simulink model "APFC_finalmodel"  (R2024b)
settings: Solver=VariableStepAuto  StartTime=0.0  StopTime=50  RelTol=1e-3
libraries: spsBreakerLib x7, spsSeriesRLCLoadLib x7, spsRMSLib x2, spsACVoltageSourceLib x1, spsCurrentMeasurementLib x1, spsVoltageMeasurementLib x1, spsMeanLib x1, spsPowerLib x1, sps_lib x1
settings Model: Creator=VICTUS  LastModifiedBy=niranjan

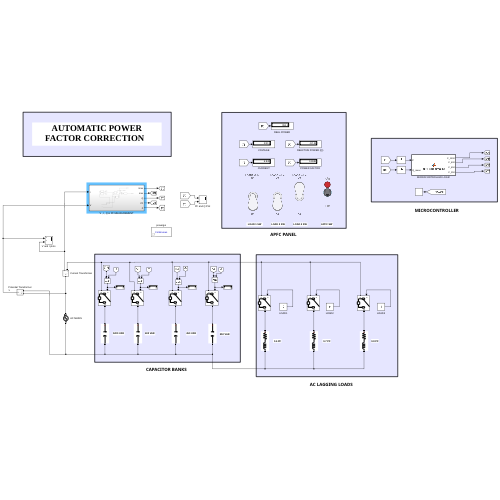
[thumbnail: Simulink's stored preview of the top-level diagram]
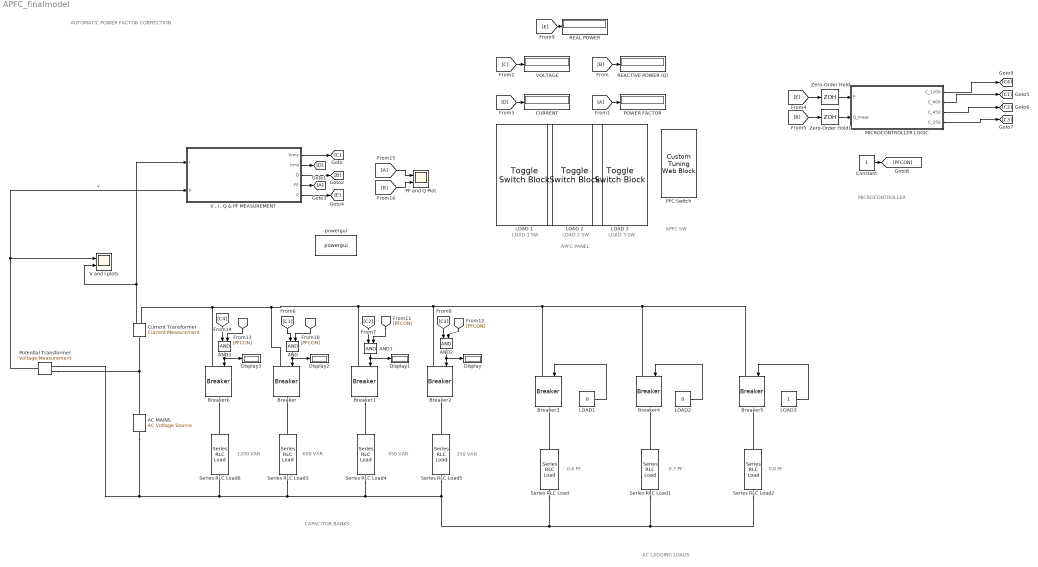
== system APFC_finalmodel ==
  note: AUTOMATIC POWER FACTOR CORRECTION
  note: CAPACITOR BANKS
  note: AC LAGGING LOADS
  note: 1200 VAR
  note: 600 VAR
  note: 450 VAR
  note: 350 VAR
  note: 0.6 PF
  note: 0.7 PF
  note: 0.8 PF
  note: MICROCONTROLLER
  note: APFC SW
  note: LOAD 3 SW
  note: LOAD 2 SW
  note: LOAD 1 SW
  note: APFC PANEL
  AC MAINS : spsACVoltageSourceLib/AC Voltage Source  Amplitude=325.27  Phase=0  Frequency=50  SampleTime=0  Measurements=None  BusType=swing  Pref=10e3  Qref=0  Qmin=-inf  Qmax=+inf
  AND{,1..3} (4 alike) : Logic  AllPortsSameDT=off  OutDataTypeStr=boolean
  Breaker{,1..6} (7 alike) : spsBreakerLib/Breaker  InitialState=0  SwitchingTimes="[1/60  5/60]"  External=on  BreakerResistance=0.01  SnubberResistance=1e6  SnubberCapacitance=inf  Measurements=None  MoreParameters=on  NoBreakLoop=off
  CURRENT : Display
  Constant : Constant
  Current Transformer : spsCurrentMeasurementLib/Current Measurement  PhasorSimulation=off  OutputType=Complex  PSBequivalent=0
  Display{,1..3} (4 alike) : Display
  From1 : From
  From15 : From
  Goto3 : Goto
  LOAD 1 : ToggleSwitchBlock
      settings: Values={{'Off', 'On'}, [0 1]}
  LOAD 2 : ToggleSwitchBlock
      settings: Values={{'Off', 'On'}, [0 1]}
  LOAD 3 : ToggleSwitchBlock
      settings: Values={{'Off', 'On'}, [0 1]}
  LOAD1 : Constant  Value=0
  LOAD2 : Constant  Value=0
  LOAD3 : Constant
  MICROCONTROLLER LOGIC : MATLAB Function  TreatAsAtomicUnit=on
  PF and Q Plot : Scope  NumInputPorts=2
  PFC Switch : CustomTuningWebBlock  LabelPosition=Hide  ShowInitialText=on  Configuration="{\"components\":[{\"name\":\"CustomSwitchStateComponent\",\"settings\":{\"position\":[0,0,1,1],\"showAllLabels\":1,\"states\":[{\"HitRegion\":{\"position\":[0.5,0,1,0.5]},\"Image\":{\"position\":[0,0.24928571428571428,0.5014285714285714,1],\"size\":[0.5014285714285714,1],\"src\":\"data:image\\/svg+xml;base64,PHN2ZyB4bWxucz0iaHR0cDovL3d3dy53My5vcmcvMjAwMC9zdmciIHhtbG5zOnhsaW5rPSJodHRwOi8vd3d3LnczLm9yZy8xOTk5L3hsaW5rIiB2aWV3Qm94PSIwIDAgMzguMDQgMTUwIj48ZGVmcz48c3R5bGU+LmNscy0xe2ZpbGw6dXJsKCNyYWRpYWwtZ3JhZGllbnQpO30uY2xzLTJ7ZmlsbDp1cmwoI3JhZGlhbC1ncmFkaWVudC0yKTt9LmNscy0ze2ZpbGw6dXJsKCNXaGl0ZV9CbGFjayk7fS5jbHMtNHtmaWxsOnVybCgjcmFkaWFsLWdyYWRpZW50LTMpO30uY2xzLTV7ZmlsbDojNWI1YjViO30uY2xzLTZ7ZmlsbDp1cmwoI3Jh ...(+3556 chars)\",\"srcOrientation\":\"Right\"},\"Label\":{\"color\":[0.5019607843137255,0.5019607843137255,0.5019607843137255],\"icon\":{\"size\":[0,0],\"src\":[],\"srcOrientation\":\"Right\"},\"iconOffset\":0,\"iconPlacement\":\"left\",\"opacity\":1,\"position\":[0.92,0.5],\"show\":true,\"text\":{\"content\":\"Off\",\"font\":\"Helvetica\"}},\"Value\":0},{\"HitRegion\":{\"position\":[0,0,1,0.5]},\"Image\":{\"position\":[0,0.24928571428571428,0.5014285714285714,1],\"size\":[0.5014285714285714,1],\"src\":\"data:image\\/svg+xml;base64,PHN2ZyB4bWxucz0iaHR0cDovL3d3dy53My5vcmcvMjAwMC9zdmciIHhtbG5zOnhsaW5rPSJodHRwOi8vd3d3LnczLm9yZy8xOTk5L3hsaW5rIiB2aWV3Qm94PSIwIDAgMzguMDQgMTUwIj48ZGVmcz48c3R5bGU+LmNscy0xe2ZpbGw6dXJsKCNyYWRpYWwtZ3JhZGllbnQpO30uY2xzLTJ7ZmlsbDp1cmwoI3JhZGlhbC1ncmFkaWVudC0yKTt9LmNscy0ze2ZpbGw6dXJsKCNXaGl0ZV9CbGFjayk7fS5jbHMtNHtmaWxsOnVybCgjcmFkaWFsLWdyYWRpZW50LTMpO30uY2xzLTV7ZmlsbDojNWI1YjViO30uY2xzLTZ7ZmlsbDp1cmwoI3Jh ...(+3628 chars)\",\"srcOrientation\":\"Right\"},\"Label\":{\"color\":[0.5019607843137255,0.5019607843137255,0.5019607843137255],\"icon\":{\"size\":[0,0],\"src\":[],\"srcOrientation\":\"Right\"},\"iconOffset\":0,\"iconPlacement\":\"left\",\"opacity\":1,\"position\":[0.08,0.5],\"show\":true,\"text\":{\"content\":\"On\",\"font\":\"Helvetica\"}},\"Value\":1}]}},{\"name\":\"BackgroundImageComponent\",\"settings\":{\"image\":{\"size\":[70,135],\"src\":\"default\",\"srcOrientation\":\"Right\"},\"position\":[0,0,1,1],\"scaleMode\":\"0\"}},{\"name\":\"ForegroundImageComponent\",\"settings\":{\"image\":{\"size\":[0,0],\"src\":\"default\",\"srcOrientation\":[]},\"isForeground\":1,\"position\":[0,0,1,1],\"scaleMode\":\"0\"}}],\"settings\":{\"BindingType\":\"param\",\"backgroundColor\":[0,0,0],\"backgroundOffset\":0.14,\"fixedAspectRatio\":\"on\",\"foregroundColor\":[0,0,0],\"showBackgroundColor\":false,\"variant\":\"toggle\",\"version\":\"R2024b\"},\"type\":\"Switch\"}"
  POWER FACTOR : Display
  Potential Transformer : spsVoltageMeasurementLib/Voltage Measurement  PhasorSimulation=off  OutputType=Complex  PSBequivalent=0
  REACTIVE POWER (Q) : Display
  REAL POWER : Display
  Series RLC Load : spsSeriesRLCLoadLib/Series RLC Load  LConnTagsString=a  RConnTagsString=__new0  NominalVoltage=230  NominalFrequency=50  ActivePower=1000  InductivePower=1333.3334  CapacitivePower=0  Setx0=off  InitialVoltage=0  SetiL0=off  InitialCurrent=0  Measurements=None  LoadType=constant Z
  Series RLC Load1 : spsSeriesRLCLoadLib/Series RLC Load  LConnTagsString=a  RConnTagsString=__new0  NominalVoltage=230  NominalFrequency=50  ActivePower=1000  InductivePower=963.8529  CapacitivePower=0  Setx0=off  InitialVoltage=0  SetiL0=off  InitialCurrent=0  Measurements=None  LoadType=constant Z
  Series RLC Load2 : spsSeriesRLCLoadLib/Series RLC Load  LConnTagsString=a  RConnTagsString=__new0  NominalVoltage=230  NominalFrequency=50  ActivePower=1000  InductivePower=750  CapacitivePower=0  Setx0=off  InitialVoltage=0  SetiL0=off  InitialCurrent=0  Measurements=None  LoadType=constant Z
  Series RLC Load3 : spsSeriesRLCLoadLib/Series RLC Load  LConnTagsString=a  RConnTagsString=__new0  NominalVoltage=230  NominalFrequency=50  ActivePower=0  InductivePower=0  CapacitivePower=600  Setx0=off  InitialVoltage=0  SetiL0=off  InitialCurrent=0  Measurements=None  LoadType=constant Z
  Series RLC Load4 : spsSeriesRLCLoadLib/Series RLC Load  LConnTagsString=a  RConnTagsString=__new0  NominalVoltage=230  NominalFrequency=50  ActivePower=0  InductivePower=0  CapacitivePower=450  Setx0=off  InitialVoltage=0  SetiL0=off  InitialCurrent=0  Measurements=None  LoadType=constant Z
  Series RLC Load5 : spsSeriesRLCLoadLib/Series RLC Load  LConnTagsString=a  RConnTagsString=__new0  NominalVoltage=230  NominalFrequency=50  ActivePower=0  InductivePower=0  CapacitivePower=350  Setx0=off  InitialVoltage=0  SetiL0=off  InitialCurrent=0  Measurements=None  LoadType=constant Z
  Series RLC Load6 : spsSeriesRLCLoadLib/Series RLC Load  LConnTagsString=a  RConnTagsString=__new0  NominalVoltage=230  NominalFrequency=50  ActivePower=0  InductivePower=0  CapacitivePower=1200  Setx0=off  InitialVoltage=0  SetiL0=off  InitialCurrent=0  Measurements=None  LoadType=constant Z
  "V , I , Q & PF MEASUREMENT" : Subsystem
  V and I plots : Scope  NumInputPorts=2
  VOLTAGE : Display
  Zero-Order Hold : ZeroOrderHold  SampleTime=10e-2
  Zero-Order Hold1 : ZeroOrderHold  SampleTime=10e-2
  powergui : sps_lib/powergui  Priority=1  SimulationMode=Continuous  SampleTime=50e-6  frequency=50  Iterations=50  frequencyindice=50  Pbase=100e6  ErrMax=1e-4  UnitsV=kV  UnitsW=MW  buscounter=0  FunctionMessages=off  echomessages=off  EnableUseOfTLC=off  CurrentSourceSwitches=off  DisableSnubberDevices=off  DisableRonSwitches=off  DisableVfSwitches=off  DisplayEquations=off  AutomaticDiscreteSolvers=off  SolverType=Tustin/Backward Euler (TBE)  Interpol=off  ExternalGateDelay=off  methode=off  Ts=100  x0status=blocks  SPID=on  SwTol=0  HookPort=off  NonlinearTolerance=1e-4  nMaxIteration=100  ContinueOnMaxIteration=off  RestoreLinks=warning  ResistiveCurrentMeasurement=off  Frange=[0:2:500]  Ylog=off  Xlog=on  ShowGrid=off  save=off  variable=ZData  structure=0  ZoomFFT=off  StartTime=0.0  cycles=1  DisplayStyle=1  fundamental=60  FreqAxis=off  MaxFrequency=1000  frequencyindicesteady=1  RmsSteady=1  display=off
  wires:
  LOAD1/1 -> Breaker3/1
  LOAD2/1 -> Breaker4/1
  LOAD3/1 -> Breaker5/1
  [B] -> REACTIVE POWER (Q)/1
  From1/1 -> POWER FACTOR/1
  [C] -> VOLTAGE/1
  [D] -> CURRENT/1
  Current Transformer/1 -> V and I plots/2, "V , I , Q & PF MEASUREMENT"/1(I)
  Potential Transformer/1 -> "V , I , Q & PF MEASUREMENT"/2(V), V and I plots/1  "V"
  "V , I , Q & PF MEASUREMENT"/1(Vrms) -> [C]
  "V , I , Q & PF MEASUREMENT"/2(Irms) -> [D]
  "V , I , Q & PF MEASUREMENT"/3(Q) -> [B]
  "V , I , Q & PF MEASUREMENT"/5(P) -> [E]
  [E] -> Zero-Order Hold/1
  [B] -> Zero-Order Hold1/1
  MICROCONTROLLER LOGIC/2(C_600) -> [C1]
  MICROCONTROLLER LOGIC/3(C_450) -> [C2]
  MICROCONTROLLER LOGIC/4(C_350) -> [C3]
  [E] -> REAL POWER/1
  "V , I , Q & PF MEASUREMENT"/4(PF) -> Goto3/1
  Constant/1 -> [PFCON]
  [C1] -> AND/1
  AND/1 -> Display2/1, Breaker/1
  AND1/1 -> Display1/1, Breaker1/1
  [C2] -> AND1/1
  [C3] -> AND2/1
  AND2/1 -> Display/1, Breaker2/1
  [PFCON] -> AND/2
  [PFCON] -> AND1/2
  [PFCON] -> AND2/2
  [C4] -> AND3/1
  [PFCON] -> AND3/2
  AND3/1 -> Display3/1, Breaker6/1
  MICROCONTROLLER LOGIC/1(C_1200) -> [C4]
  From15/1 -> PF and Q Plot/1
  Zero-Order Hold/1 -> MICROCONTROLLER LOGIC/1(P)
  Zero-Order Hold1/1 -> MICROCONTROLLER LOGIC/2(Q_meas)
  [B] -> PF and Q Plot/2
  connections:
  Series RLC Load/RConn1 -- Series RLC Load2/RConn1 -- Series RLC Load1/RConn1 -- Series RLC Load5/RConn1 -- Potential Transformer/LConn2 -- AC MAINS/LConn1 -- Series RLC Load6/RConn1 -- Series RLC Load3/RConn1 -- Series RLC Load4/RConn1
  Breaker/LConn1 -- Breaker1/LConn1 -- Breaker2/LConn1 -- Breaker3/LConn1 -- Breaker4/LConn1 -- Breaker5/LConn1 -- Breaker6/LConn1 -- Current Transformer/RConn1
  AC MAINS/RConn1 -- Potential Transformer/LConn1 -- Current Transformer/LConn1
  Series RLC Load/LConn1 -- Breaker3/RConn1
  Series RLC Load1/LConn1 -- Breaker4/RConn1
  Series RLC Load2/LConn1 -- Breaker5/RConn1
  Series RLC Load3/LConn1 -- Breaker/RConn1
  Breaker2/RConn1 -- Series RLC Load5/LConn1
  Breaker1/RConn1 -- Series RLC Load4/LConn1
  Breaker6/RConn1 -- Series RLC Load6/LConn1

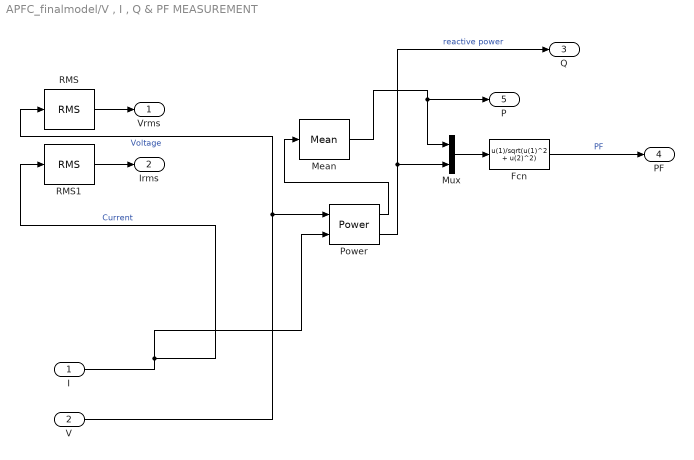
== system APFC_finalmodel/V , I , Q & PF MEASUREMENT ==
  I : Inport
  V : Inport  Port=2
  Fcn : Fcn  Expr=u(1)/sqrt(u(1)^2 + u(2)^2)
  Mean : spsMeanLib/Mean  Freq=50  Vinit=0  Ts=0
  Mux : Mux  Inputs=2
  Power : spsPowerLib/Power  Freq=50  Vinit=[0 0]  Iinit=[0, 0]  Ts=0
  RMS : spsRMSLib/RMS  TrueRMS=on  Freq=50  RMSInit=0  Ts=0
  RMS1 : spsRMSLib/RMS  TrueRMS=on  Freq=50  RMSInit=0  Ts=0
  Vrms : Outport
  Irms : Outport  Port=2
  Q : Outport  Port=3
  PF : Outport  Port=4
  P : Outport  Port=5
  wires:
  Mux/1 -> Fcn/1
  I/1 -> Power/2, RMS1/1  "Current"
  V/1 -> RMS/1, Power/1  "Voltage"
  RMS/1 -> Vrms/1
  RMS1/1 -> Irms/1
  Power/1 -> Mean/1
  Mean/1 -> Mux/1, P/1
  Fcn/1 -> PF/1  "PF"
  Power/2 -> Q/1, Mux/2  "reactive power"

== matlab function APFC_finalmodel/MICROCONTROLLER LOGIC ==
  settings: updateMethod=DISCRETE
  data: C_1200 output; P input; C_600 output; Q_meas input; C_450 output; C_350 output
function [C_1200, C_600, C_450, C_350] = apfc_logic_simulink(P, Q_meas)
    
    % 1. Memory of Current State
    % Update the persistent array to hold 4 states instead of 3
    persistent current_caps;
    if isempty(current_caps)
        current_caps = [0, 0, 0, 0];
    end
    
    % 2. Configuration
    % Add your new 1200 VAR bank to the front
    caps = [1200, 600, 450, 350];
    n = length(caps);
    
    % 3. RECONSTRUCT THE TRUE LOAD
    % True Load = Measured Grid Q + Q currently supplied by our capacitors
    Q_active = sum(current_caps .* caps);
    Q_load = Q_meas + Q_active; 
    
    % 4. Safety Deadband (Based on the TRUE load)
    S_load = sqrt(P^2 + Q_load^2); 
    if S_load < 100 || abs(Q_load) < 50
        current_caps = [0, 0, 0, 0];
        C_1200 = 0; C_600 = 0; C_450 = 0; C_350 = 0;
        return;
    end
    
    % 5. Generate all combinations (Automatically handles 16 states)
    num_combos = 2^n;
    combos = zeros(num_combos, n);
    total_q_cap = zeros(num_combos, 1);
    
    for i = 0:num_combos-1
        bits = bitget(i, n:-1:1); 
        combos(i+1, :) = bits;
        total_q_cap(i+1) = sum(bits .* caps);
    end
    
    % 6. Calculate cost against the TRUE LOAD (Q_load)
    q_remaining = Q_load - total_q_cap;
    cost = abs(q_remaining);
    cost(q_remaining < 0) = cost(q_remaining < 0) * 1.2; % Penalty for over-compensation
    
    % 7. Calculate the cost of our CURRENT state
    current_q_rem = Q_load - Q_active;
    current_cost = abs(current_q_rem);
    if current_q_rem < 0
        current_cost = current_cost * 1.2;
    end
    
    % 8. Hysteresis Decision Logic
    % Find the best possible combination
    [min_cost, best_idx] = min(cost);
    best_caps = combos(best_idx, :);
    
    % Only switch if the new combination is at least 100 VAR better than staying put
    hysteresis_band = 100; 
    if (current_cost - min_cost) > hysteresis_band
        current_caps = best_caps; 
    end
    
    % 9. Assign Outputs
    C_1200 = current_caps(1);
    C_600  = current_caps(2);
    C_450  = current_caps(3);
    C_350  = current_caps(4);
end
